simulink model "CartPend_simul"  (R2017a)
settings: Solver=VariableStepAuto  StartTime=0.0  StopTime=10.0  RelTol=1e-3
values from neighbouring files (symbols this model uses):
  A = [0      1              0           0 ... (first row only)    [CartPend_main.m]
  B = [     0 ... (first row only)    [CartPend_main.m]
  C = [1 0 0 0 ... (first row only)    [CartPend_main.m]
  D = [0 ... (first row only)    [CartPend_main.m]    (also in PlotTanks.m = 40)
undefined symbols (not defined in the file or in its folder): DC_gain, Dis_instant, Dis_interval, Dis_size, K, L
settings Model: Creator=root  LastModifiedBy=root

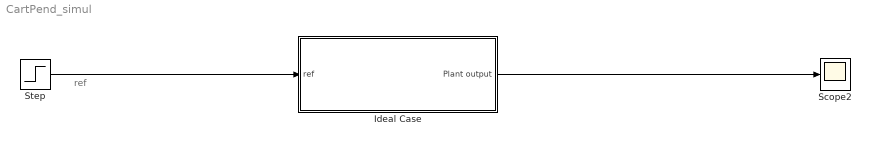
== system CartPend_simul ==
  note: ref
  Ideal Case : Subsystem
  Scope2 : Scope
  Step : Step  Time=0  After=1/DC_gain  SampleTime=0
  wires:
  Step/1 -> Ideal Case/1(ref)
  Ideal Case/1(Plant output) -> Scope2/1

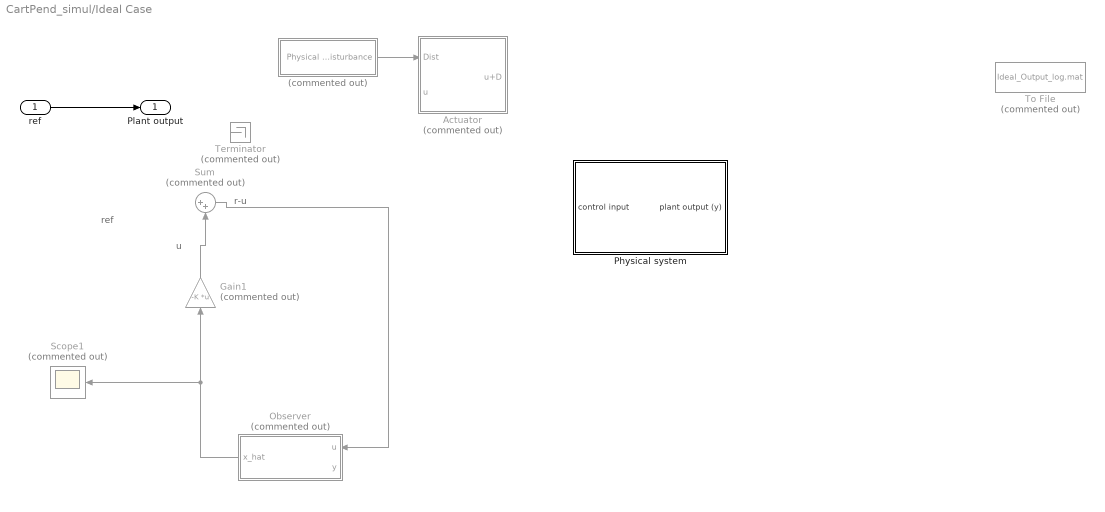
== system CartPend_simul/Ideal Case ==
  note: u
  note: ref
  note: r-u
  ref : Inport
  " " : Subsystem  Commented=on
  Actuator : Subsystem  Commented=on
  Gain1 : Gain  Commented=on  Gain=-K  Multiplication=Matrix(K*u)
  Observer : Subsystem  Commented=on
  Physical system : Subsystem
  Scope1 : Scope  Commented=on
  Sum : Sum  Commented=on  Inputs=|++
  Terminator : Terminator  Commented=on
  To File : ToFile  Commented=on  Filename=Ideal_Output_log.mat  SaveFormat=Timeseries
  Plant output : Outport
  wires:
  Observer/1(x_hat) -> Scope1/1, Gain1/1
  Gain1/1 -> Sum/2
  Sum/1 -> Observer/1(u)
  " "/1(Physical Disturbance) -> Actuator/1(Dist)
  ref/1 -> Plant output/1

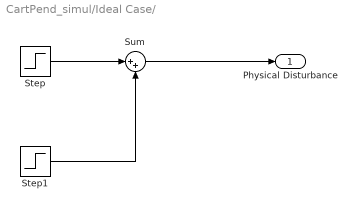
== system CartPend_simul/Ideal Case/  ==
  Step : Step  Time=Dis_instant  After=Dis_size  SampleTime=0
  Step1 : Step  Time=Dis_instant+Dis_interval  After=-Dis_size  SampleTime=0
  Sum : Sum  Inputs=|++
  Physical Disturbance : Outport
  wires:
  Step/1 -> Sum/1
  Step1/1 -> Sum/2
  Sum/1 -> Physical Disturbance/1

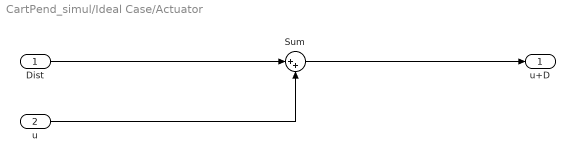
== system CartPend_simul/Ideal Case/Actuator ==
  Dist : Inport
  u : Inport  Port=2
  Sum : Sum  Inputs=|++
  u+D : Outport
  wires:
  u/1 -> Sum/2
  Dist/1 -> Sum/1
  Sum/1 -> u+D/1

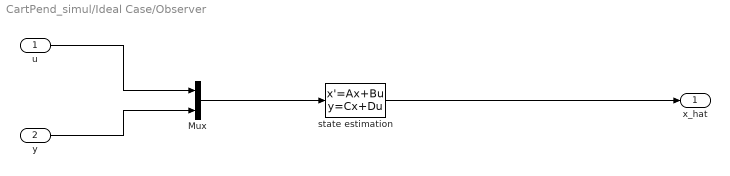
== system CartPend_simul/Ideal Case/Observer ==
  u : Inport
  y : Inport  Port=2
  Mux : Mux  Inputs=2
  "state estimation " : StateSpace  A=A-L*C  B=[B L]  C=eye(2)  D=[0 0;0 0]  X0=0
  x_hat : Outport
  wires:
  u/1 -> Mux/1
  y/1 -> Mux/2
  Mux/1 -> "state estimation "/1
  "state estimation "/1 -> x_hat/1

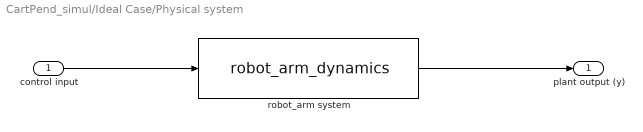
== system CartPend_simul/Ideal Case/Physical system ==
  control input : Inport
  robot_arm system : S-Function  FunctionName=robot_arm_dynamics  Parameters=A,B,C,D  SFunctionDeploymentMode=off  EnableBusSupport=off
  plant output (y) : Outport
  wires:
  control input/1 -> robot_arm system/1
  robot_arm system/1 -> plant output (y)/1
